simulink model "MdXX_RspOutComm"  (R2022b)
settings: Solver=FixedStepDiscrete  StartTime=0.0  StopTime=10.0  FixedStep=0.01  RelTol=1e-3
undefined symbols (not defined in the file or in its folder): KeSMSuRspStatHldTm_Val, MdRspLocal2, SrcReqTp1
libraries: simulink x64, RspLib x32
(part 4 of 5)

== system MdXX_RspOutComm/MdXX_RspOutCommCalc_Cal_sys/Subsystem/MdRspOutDataSelc13/BitSelector ==
  U : Inport
  Bit : Inport  Port=2
  Bitwise Operator : simulink/Logic and Bit Operations/Bitwise Operator  logicop=AND  UseBitMask=off  NumInputPorts=2  BitMask=bin2dec('11011001')  BitMaskRealWorld=Stored Integer
  Constant2 : Constant  OutDataTypeStr=uint32
  Constant4 : Constant  Value=0  OutDataTypeStr=uint32
  Relational Operator : RelationalOperator  Operator=>  OutDataTypeStr=boolean  RndMeth=Simplest  InputSameDT=off
  Shift Arithmetic : ArithShift  BitShiftNumberSource=Input port  BitShiftNumber=8  BitShiftDirection=Left
      settings: InputPortMap=u0,p1
  BitOut : Outport  VectorParamsAs1DForOutWhenUnconnected=off
  wires:
  Relational Operator/1 -> BitOut/1
  Constant4/1 -> Relational Operator/2
  Constant2/1 -> Shift Arithmetic/1
  Bitwise Operator/1 -> Relational Operator/1
  U/1 -> Bitwise Operator/1
  Shift Arithmetic/1 -> Bitwise Operator/2
  Bit/1 -> Shift Arithmetic/2

== system MdXX_RspOutComm/MdXX_RspOutCommCalc_Cal_sys/Subsystem/MdRspOutDataSelc13/BitSelector1 ==
  U : Inport
  Bit : Inport  Port=2
  Bitwise Operator : simulink/Logic and Bit Operations/Bitwise Operator  logicop=AND  UseBitMask=off  NumInputPorts=2  BitMask=bin2dec('11011001')  BitMaskRealWorld=Stored Integer
  Constant2 : Constant  OutDataTypeStr=uint32
  Constant4 : Constant  Value=0  OutDataTypeStr=uint32
  Relational Operator : RelationalOperator  Operator=>  OutDataTypeStr=boolean  RndMeth=Simplest  InputSameDT=off
  Shift Arithmetic : ArithShift  BitShiftNumberSource=Input port  BitShiftNumber=8  BitShiftDirection=Left
      settings: InputPortMap=u0,p1
  BitOut : Outport  VectorParamsAs1DForOutWhenUnconnected=off
  wires:
  Bit/1 -> Shift Arithmetic/2
  Shift Arithmetic/1 -> Bitwise Operator/2
  U/1 -> Bitwise Operator/1
  Bitwise Operator/1 -> Relational Operator/1
  Constant2/1 -> Shift Arithmetic/1
  Constant4/1 -> Relational Operator/2
  Relational Operator/1 -> BitOut/1

== system MdXX_RspOutComm/MdXX_RspOutCommCalc_Cal_sys/Subsystem/MdRspOutDataSelc14/BitSelector ==
  U : Inport
  Bit : Inport  Port=2
  Bitwise Operator : simulink/Logic and Bit Operations/Bitwise Operator  logicop=AND  UseBitMask=off  NumInputPorts=2  BitMask=bin2dec('11011001')  BitMaskRealWorld=Stored Integer
  Constant2 : Constant  OutDataTypeStr=uint32
  Constant4 : Constant  Value=0  OutDataTypeStr=uint32
  Relational Operator : RelationalOperator  Operator=>  OutDataTypeStr=boolean  RndMeth=Simplest  InputSameDT=off
  Shift Arithmetic : ArithShift  BitShiftNumberSource=Input port  BitShiftNumber=8  BitShiftDirection=Left
      settings: InputPortMap=u0,p1
  BitOut : Outport  VectorParamsAs1DForOutWhenUnconnected=off
  wires:
  Bit/1 -> Shift Arithmetic/2
  Shift Arithmetic/1 -> Bitwise Operator/2
  U/1 -> Bitwise Operator/1
  Bitwise Operator/1 -> Relational Operator/1
  Constant2/1 -> Shift Arithmetic/1
  Constant4/1 -> Relational Operator/2
  Relational Operator/1 -> BitOut/1

== system MdXX_RspOutComm/MdXX_RspOutCommCalc_Cal_sys/Subsystem/MdRspOutDataSelc14/BitSelector1 ==
  U : Inport
  Bit : Inport  Port=2
  Bitwise Operator : simulink/Logic and Bit Operations/Bitwise Operator  logicop=AND  UseBitMask=off  NumInputPorts=2  BitMask=bin2dec('11011001')  BitMaskRealWorld=Stored Integer
  Constant2 : Constant  OutDataTypeStr=uint32
  Constant4 : Constant  Value=0  OutDataTypeStr=uint32
  Relational Operator : RelationalOperator  Operator=>  OutDataTypeStr=boolean  RndMeth=Simplest  InputSameDT=off
  Shift Arithmetic : ArithShift  BitShiftNumberSource=Input port  BitShiftNumber=8  BitShiftDirection=Left
      settings: InputPortMap=u0,p1
  BitOut : Outport  VectorParamsAs1DForOutWhenUnconnected=off
  wires:
  Relational Operator/1 -> BitOut/1
  Constant4/1 -> Relational Operator/2
  Constant2/1 -> Shift Arithmetic/1
  Bitwise Operator/1 -> Relational Operator/1
  U/1 -> Bitwise Operator/1
  Shift Arithmetic/1 -> Bitwise Operator/2
  Bit/1 -> Shift Arithmetic/2

== system MdXX_RspOutComm/MdXX_RspOutCommCalc_Cal_sys/Subsystem/MdRspOutDataSelc15/BitSelector ==
  U : Inport
  Bit : Inport  Port=2
  Bitwise Operator : simulink/Logic and Bit Operations/Bitwise Operator  logicop=AND  UseBitMask=off  NumInputPorts=2  BitMask=bin2dec('11011001')  BitMaskRealWorld=Stored Integer
  Constant2 : Constant  OutDataTypeStr=uint32
  Constant4 : Constant  Value=0  OutDataTypeStr=uint32
  Relational Operator : RelationalOperator  Operator=>  OutDataTypeStr=boolean  RndMeth=Simplest  InputSameDT=off
  Shift Arithmetic : ArithShift  BitShiftNumberSource=Input port  BitShiftNumber=8  BitShiftDirection=Left
      settings: InputPortMap=u0,p1
  BitOut : Outport  VectorParamsAs1DForOutWhenUnconnected=off
  wires:
  Relational Operator/1 -> BitOut/1
  Constant4/1 -> Relational Operator/2
  Constant2/1 -> Shift Arithmetic/1
  Bitwise Operator/1 -> Relational Operator/1
  U/1 -> Bitwise Operator/1
  Shift Arithmetic/1 -> Bitwise Operator/2
  Bit/1 -> Shift Arithmetic/2

== system MdXX_RspOutComm/MdXX_RspOutCommCalc_Cal_sys/Subsystem/MdRspOutDataSelc15/BitSelector1 ==
  U : Inport
  Bit : Inport  Port=2
  Bitwise Operator : simulink/Logic and Bit Operations/Bitwise Operator  logicop=AND  UseBitMask=off  NumInputPorts=2  BitMask=bin2dec('11011001')  BitMaskRealWorld=Stored Integer
  Constant2 : Constant  OutDataTypeStr=uint32
  Constant4 : Constant  Value=0  OutDataTypeStr=uint32
  Relational Operator : RelationalOperator  Operator=>  OutDataTypeStr=boolean  RndMeth=Simplest  InputSameDT=off
  Shift Arithmetic : ArithShift  BitShiftNumberSource=Input port  BitShiftNumber=8  BitShiftDirection=Left
      settings: InputPortMap=u0,p1
  BitOut : Outport  VectorParamsAs1DForOutWhenUnconnected=off
  wires:
  Bit/1 -> Shift Arithmetic/2
  Shift Arithmetic/1 -> Bitwise Operator/2
  U/1 -> Bitwise Operator/1
  Bitwise Operator/1 -> Relational Operator/1
  Constant2/1 -> Shift Arithmetic/1
  Constant4/1 -> Relational Operator/2
  Relational Operator/1 -> BitOut/1

== system MdXX_RspOutComm/MdXX_RspOutCommCalc_Cal_sys/Subsystem/MdRspOutDataSelc16/BitSelector ==
  U : Inport
  Bit : Inport  Port=2
  Bitwise Operator : simulink/Logic and Bit Operations/Bitwise Operator  logicop=AND  UseBitMask=off  NumInputPorts=2  BitMask=bin2dec('11011001')  BitMaskRealWorld=Stored Integer
  Constant2 : Constant  OutDataTypeStr=uint32
  Constant4 : Constant  Value=0  OutDataTypeStr=uint32
  Relational Operator : RelationalOperator  Operator=>  OutDataTypeStr=boolean  RndMeth=Simplest  InputSameDT=off
  Shift Arithmetic : ArithShift  BitShiftNumberSource=Input port  BitShiftNumber=8  BitShiftDirection=Left
      settings: InputPortMap=u0,p1
  BitOut : Outport  VectorParamsAs1DForOutWhenUnconnected=off
  wires:
  Bit/1 -> Shift Arithmetic/2
  Shift Arithmetic/1 -> Bitwise Operator/2
  U/1 -> Bitwise Operator/1
  Bitwise Operator/1 -> Relational Operator/1
  Constant2/1 -> Shift Arithmetic/1
  Constant4/1 -> Relational Operator/2
  Relational Operator/1 -> BitOut/1

== system MdXX_RspOutComm/MdXX_RspOutCommCalc_Cal_sys/Subsystem/MdRspOutDataSelc16/BitSelector1 ==
  U : Inport
  Bit : Inport  Port=2
  Bitwise Operator : simulink/Logic and Bit Operations/Bitwise Operator  logicop=AND  UseBitMask=off  NumInputPorts=2  BitMask=bin2dec('11011001')  BitMaskRealWorld=Stored Integer
  Constant2 : Constant  OutDataTypeStr=uint32
  Constant4 : Constant  Value=0  OutDataTypeStr=uint32
  Relational Operator : RelationalOperator  Operator=>  OutDataTypeStr=boolean  RndMeth=Simplest  InputSameDT=off
  Shift Arithmetic : ArithShift  BitShiftNumberSource=Input port  BitShiftNumber=8  BitShiftDirection=Left
      settings: InputPortMap=u0,p1
  BitOut : Outport  VectorParamsAs1DForOutWhenUnconnected=off
  wires:
  Relational Operator/1 -> BitOut/1
  Constant4/1 -> Relational Operator/2
  Constant2/1 -> Shift Arithmetic/1
  Bitwise Operator/1 -> Relational Operator/1
  U/1 -> Bitwise Operator/1
  Shift Arithmetic/1 -> Bitwise Operator/2
  Bit/1 -> Shift Arithmetic/2

== system MdXX_RspOutComm/MdXX_RspOutCommCalc_Cal_sys/Subsystem/MdRspOutDataSelc17/BitSelector ==
  U : Inport
  Bit : Inport  Port=2
  Bitwise Operator : simulink/Logic and Bit Operations/Bitwise Operator  logicop=AND  UseBitMask=off  NumInputPorts=2  BitMask=bin2dec('11011001')  BitMaskRealWorld=Stored Integer
  Constant2 : Constant  OutDataTypeStr=uint32
  Constant4 : Constant  Value=0  OutDataTypeStr=uint32
  Relational Operator : RelationalOperator  Operator=>  OutDataTypeStr=boolean  RndMeth=Simplest  InputSameDT=off
  Shift Arithmetic : ArithShift  BitShiftNumberSource=Input port  BitShiftNumber=8  BitShiftDirection=Left
      settings: InputPortMap=u0,p1
  BitOut : Outport  VectorParamsAs1DForOutWhenUnconnected=off
  wires:
  Relational Operator/1 -> BitOut/1
  Constant4/1 -> Relational Operator/2
  Constant2/1 -> Shift Arithmetic/1
  Bitwise Operator/1 -> Relational Operator/1
  U/1 -> Bitwise Operator/1
  Shift Arithmetic/1 -> Bitwise Operator/2
  Bit/1 -> Shift Arithmetic/2

== system MdXX_RspOutComm/MdXX_RspOutCommCalc_Cal_sys/Subsystem/MdRspOutDataSelc17/BitSelector1 ==
  U : Inport
  Bit : Inport  Port=2
  Bitwise Operator : simulink/Logic and Bit Operations/Bitwise Operator  logicop=AND  UseBitMask=off  NumInputPorts=2  BitMask=bin2dec('11011001')  BitMaskRealWorld=Stored Integer
  Constant2 : Constant  OutDataTypeStr=uint32
  Constant4 : Constant  Value=0  OutDataTypeStr=uint32
  Relational Operator : RelationalOperator  Operator=>  OutDataTypeStr=boolean  RndMeth=Simplest  InputSameDT=off
  Shift Arithmetic : ArithShift  BitShiftNumberSource=Input port  BitShiftNumber=8  BitShiftDirection=Left
      settings: InputPortMap=u0,p1
  BitOut : Outport  VectorParamsAs1DForOutWhenUnconnected=off
  wires:
  Bit/1 -> Shift Arithmetic/2
  Shift Arithmetic/1 -> Bitwise Operator/2
  U/1 -> Bitwise Operator/1
  Bitwise Operator/1 -> Relational Operator/1
  Constant2/1 -> Shift Arithmetic/1
  Constant4/1 -> Relational Operator/2
  Relational Operator/1 -> BitOut/1

== system MdXX_RspOutComm/MdXX_RspOutCommCalc_Cal_sys/Subsystem/MdRspOutDataSelc18/BitSelector ==
  U : Inport
  Bit : Inport  Port=2
  Bitwise Operator : simulink/Logic and Bit Operations/Bitwise Operator  logicop=AND  UseBitMask=off  NumInputPorts=2  BitMask=bin2dec('11011001')  BitMaskRealWorld=Stored Integer
  Constant2 : Constant  OutDataTypeStr=uint32
  Constant4 : Constant  Value=0  OutDataTypeStr=uint32
  Relational Operator : RelationalOperator  Operator=>  OutDataTypeStr=boolean  RndMeth=Simplest  InputSameDT=off
  Shift Arithmetic : ArithShift  BitShiftNumberSource=Input port  BitShiftNumber=8  BitShiftDirection=Left
      settings: InputPortMap=u0,p1
  BitOut : Outport  VectorParamsAs1DForOutWhenUnconnected=off
  wires:
  Bit/1 -> Shift Arithmetic/2
  Shift Arithmetic/1 -> Bitwise Operator/2
  U/1 -> Bitwise Operator/1
  Bitwise Operator/1 -> Relational Operator/1
  Constant2/1 -> Shift Arithmetic/1
  Constant4/1 -> Relational Operator/2
  Relational Operator/1 -> BitOut/1

== system MdXX_RspOutComm/MdXX_RspOutCommCalc_Cal_sys/Subsystem/MdRspOutDataSelc18/BitSelector1 ==
  U : Inport
  Bit : Inport  Port=2
  Bitwise Operator : simulink/Logic and Bit Operations/Bitwise Operator  logicop=AND  UseBitMask=off  NumInputPorts=2  BitMask=bin2dec('11011001')  BitMaskRealWorld=Stored Integer
  Constant2 : Constant  OutDataTypeStr=uint32
  Constant4 : Constant  Value=0  OutDataTypeStr=uint32
  Relational Operator : RelationalOperator  Operator=>  OutDataTypeStr=boolean  RndMeth=Simplest  InputSameDT=off
  Shift Arithmetic : ArithShift  BitShiftNumberSource=Input port  BitShiftNumber=8  BitShiftDirection=Left
      settings: InputPortMap=u0,p1
  BitOut : Outport  VectorParamsAs1DForOutWhenUnconnected=off
  wires:
  Relational Operator/1 -> BitOut/1
  Constant4/1 -> Relational Operator/2
  Constant2/1 -> Shift Arithmetic/1
  Bitwise Operator/1 -> Relational Operator/1
  U/1 -> Bitwise Operator/1
  Shift Arithmetic/1 -> Bitwise Operator/2
  Bit/1 -> Shift Arithmetic/2

== system MdXX_RspOutComm/MdXX_RspOutCommCalc_Cal_sys/Subsystem/MdRspOutDataSelc19/BitSelector ==
  U : Inport
  Bit : Inport  Port=2
  Bitwise Operator : simulink/Logic and Bit Operations/Bitwise Operator  logicop=AND  UseBitMask=off  NumInputPorts=2  BitMask=bin2dec('11011001')  BitMaskRealWorld=Stored Integer
  Constant2 : Constant  OutDataTypeStr=uint32
  Constant4 : Constant  Value=0  OutDataTypeStr=uint32
  Relational Operator : RelationalOperator  Operator=>  OutDataTypeStr=boolean  RndMeth=Simplest  InputSameDT=off
  Shift Arithmetic : ArithShift  BitShiftNumberSource=Input port  BitShiftNumber=8  BitShiftDirection=Left
      settings: InputPortMap=u0,p1
  BitOut : Outport  VectorParamsAs1DForOutWhenUnconnected=off
  wires:
  Relational Operator/1 -> BitOut/1
  Constant4/1 -> Relational Operator/2
  Constant2/1 -> Shift Arithmetic/1
  Bitwise Operator/1 -> Relational Operator/1
  U/1 -> Bitwise Operator/1
  Shift Arithmetic/1 -> Bitwise Operator/2
  Bit/1 -> Shift Arithmetic/2

== system MdXX_RspOutComm/MdXX_RspOutCommCalc_Cal_sys/Subsystem/MdRspOutDataSelc19/BitSelector1 ==
  U : Inport
  Bit : Inport  Port=2
  Bitwise Operator : simulink/Logic and Bit Operations/Bitwise Operator  logicop=AND  UseBitMask=off  NumInputPorts=2  BitMask=bin2dec('11011001')  BitMaskRealWorld=Stored Integer
  Constant2 : Constant  OutDataTypeStr=uint32
  Constant4 : Constant  Value=0  OutDataTypeStr=uint32
  Relational Operator : RelationalOperator  Operator=>  OutDataTypeStr=boolean  RndMeth=Simplest  InputSameDT=off
  Shift Arithmetic : ArithShift  BitShiftNumberSource=Input port  BitShiftNumber=8  BitShiftDirection=Left
      settings: InputPortMap=u0,p1
  BitOut : Outport  VectorParamsAs1DForOutWhenUnconnected=off
  wires:
  Bit/1 -> Shift Arithmetic/2
  Shift Arithmetic/1 -> Bitwise Operator/2
  U/1 -> Bitwise Operator/1
  Bitwise Operator/1 -> Relational Operator/1
  Constant2/1 -> Shift Arithmetic/1
  Constant4/1 -> Relational Operator/2
  Relational Operator/1 -> BitOut/1

== system MdXX_RspOutComm/MdXX_RspOutCommCalc_Cal_sys/Subsystem/MdRspOutDataSelc2/BitSelector ==
  U : Inport
  Bit : Inport  Port=2
  Bitwise Operator : simulink/Logic and Bit Operations/Bitwise Operator  logicop=AND  UseBitMask=off  NumInputPorts=2  BitMask=bin2dec('11011001')  BitMaskRealWorld=Stored Integer
  Constant2 : Constant  OutDataTypeStr=uint32
  Constant4 : Constant  Value=0  OutDataTypeStr=uint32
  Relational Operator : RelationalOperator  Operator=>  OutDataTypeStr=boolean  RndMeth=Simplest  InputSameDT=off
  Shift Arithmetic : ArithShift  BitShiftNumberSource=Input port  BitShiftNumber=8  BitShiftDirection=Left
      settings: InputPortMap=u0,p1
  BitOut : Outport  VectorParamsAs1DForOutWhenUnconnected=off
  wires:
  Bit/1 -> Shift Arithmetic/2
  Shift Arithmetic/1 -> Bitwise Operator/2
  U/1 -> Bitwise Operator/1
  Bitwise Operator/1 -> Relational Operator/1
  Constant2/1 -> Shift Arithmetic/1
  Constant4/1 -> Relational Operator/2
  Relational Operator/1 -> BitOut/1

== system MdXX_RspOutComm/MdXX_RspOutCommCalc_Cal_sys/Subsystem/MdRspOutDataSelc2/BitSelector1 ==
  U : Inport
  Bit : Inport  Port=2
  Bitwise Operator : simulink/Logic and Bit Operations/Bitwise Operator  logicop=AND  UseBitMask=off  NumInputPorts=2  BitMask=bin2dec('11011001')  BitMaskRealWorld=Stored Integer
  Constant2 : Constant  OutDataTypeStr=uint32
  Constant4 : Constant  Value=0  OutDataTypeStr=uint32
  Relational Operator : RelationalOperator  Operator=>  OutDataTypeStr=boolean  RndMeth=Simplest  InputSameDT=off
  Shift Arithmetic : ArithShift  BitShiftNumberSource=Input port  BitShiftNumber=8  BitShiftDirection=Left
      settings: InputPortMap=u0,p1
  BitOut : Outport  VectorParamsAs1DForOutWhenUnconnected=off
  wires:
  Relational Operator/1 -> BitOut/1
  Constant4/1 -> Relational Operator/2
  Constant2/1 -> Shift Arithmetic/1
  Bitwise Operator/1 -> Relational Operator/1
  U/1 -> Bitwise Operator/1
  Shift Arithmetic/1 -> Bitwise Operator/2
  Bit/1 -> Shift Arithmetic/2

== system MdXX_RspOutComm/MdXX_RspOutCommCalc_Cal_sys/Subsystem/MdRspOutDataSelc20/BitSelector ==
  U : Inport
  Bit : Inport  Port=2
  Bitwise Operator : simulink/Logic and Bit Operations/Bitwise Operator  logicop=AND  UseBitMask=off  NumInputPorts=2  BitMask=bin2dec('11011001')  BitMaskRealWorld=Stored Integer
  Constant2 : Constant  OutDataTypeStr=uint32
  Constant4 : Constant  Value=0  OutDataTypeStr=uint32
  Relational Operator : RelationalOperator  Operator=>  OutDataTypeStr=boolean  RndMeth=Simplest  InputSameDT=off
  Shift Arithmetic : ArithShift  BitShiftNumberSource=Input port  BitShiftNumber=8  BitShiftDirection=Left
      settings: InputPortMap=u0,p1
  BitOut : Outport  VectorParamsAs1DForOutWhenUnconnected=off
  wires:
  Bit/1 -> Shift Arithmetic/2
  Shift Arithmetic/1 -> Bitwise Operator/2
  U/1 -> Bitwise Operator/1
  Bitwise Operator/1 -> Relational Operator/1
  Constant2/1 -> Shift Arithmetic/1
  Constant4/1 -> Relational Operator/2
  Relational Operator/1 -> BitOut/1

== system MdXX_RspOutComm/MdXX_RspOutCommCalc_Cal_sys/Subsystem/MdRspOutDataSelc20/BitSelector1 ==
  U : Inport
  Bit : Inport  Port=2
  Bitwise Operator : simulink/Logic and Bit Operations/Bitwise Operator  logicop=AND  UseBitMask=off  NumInputPorts=2  BitMask=bin2dec('11011001')  BitMaskRealWorld=Stored Integer
  Constant2 : Constant  OutDataTypeStr=uint32
  Constant4 : Constant  Value=0  OutDataTypeStr=uint32
  Relational Operator : RelationalOperator  Operator=>  OutDataTypeStr=boolean  RndMeth=Simplest  InputSameDT=off
  Shift Arithmetic : ArithShift  BitShiftNumberSource=Input port  BitShiftNumber=8  BitShiftDirection=Left
      settings: InputPortMap=u0,p1
  BitOut : Outport  VectorParamsAs1DForOutWhenUnconnected=off
  wires:
  Relational Operator/1 -> BitOut/1
  Constant4/1 -> Relational Operator/2
  Constant2/1 -> Shift Arithmetic/1
  Bitwise Operator/1 -> Relational Operator/1
  U/1 -> Bitwise Operator/1
  Shift Arithmetic/1 -> Bitwise Operator/2
  Bit/1 -> Shift Arithmetic/2

== system MdXX_RspOutComm/MdXX_RspOutCommCalc_Cal_sys/Subsystem/MdRspOutDataSelc21/BitSelector ==
  U : Inport
  Bit : Inport  Port=2
  Bitwise Operator : simulink/Logic and Bit Operations/Bitwise Operator  logicop=AND  UseBitMask=off  NumInputPorts=2  BitMask=bin2dec('11011001')  BitMaskRealWorld=Stored Integer
  Constant2 : Constant  OutDataTypeStr=uint32
  Constant4 : Constant  Value=0  OutDataTypeStr=uint32
  Relational Operator : RelationalOperator  Operator=>  OutDataTypeStr=boolean  RndMeth=Simplest  InputSameDT=off
  Shift Arithmetic : ArithShift  BitShiftNumberSource=Input port  BitShiftNumber=8  BitShiftDirection=Left
      settings: InputPortMap=u0,p1
  BitOut : Outport  VectorParamsAs1DForOutWhenUnconnected=off
  wires:
  Relational Operator/1 -> BitOut/1
  Constant4/1 -> Relational Operator/2
  Constant2/1 -> Shift Arithmetic/1
  Bitwise Operator/1 -> Relational Operator/1
  U/1 -> Bitwise Operator/1
  Shift Arithmetic/1 -> Bitwise Operator/2
  Bit/1 -> Shift Arithmetic/2

== system MdXX_RspOutComm/MdXX_RspOutCommCalc_Cal_sys/Subsystem/MdRspOutDataSelc21/BitSelector1 ==
  U : Inport
  Bit : Inport  Port=2
  Bitwise Operator : simulink/Logic and Bit Operations/Bitwise Operator  logicop=AND  UseBitMask=off  NumInputPorts=2  BitMask=bin2dec('11011001')  BitMaskRealWorld=Stored Integer
  Constant2 : Constant  OutDataTypeStr=uint32
  Constant4 : Constant  Value=0  OutDataTypeStr=uint32
  Relational Operator : RelationalOperator  Operator=>  OutDataTypeStr=boolean  RndMeth=Simplest  InputSameDT=off
  Shift Arithmetic : ArithShift  BitShiftNumberSource=Input port  BitShiftNumber=8  BitShiftDirection=Left
      settings: InputPortMap=u0,p1
  BitOut : Outport  VectorParamsAs1DForOutWhenUnconnected=off
  wires:
  Bit/1 -> Shift Arithmetic/2
  Shift Arithmetic/1 -> Bitwise Operator/2
  U/1 -> Bitwise Operator/1
  Bitwise Operator/1 -> Relational Operator/1
  Constant2/1 -> Shift Arithmetic/1
  Constant4/1 -> Relational Operator/2
  Relational Operator/1 -> BitOut/1

== system MdXX_RspOutComm/MdXX_RspOutCommCalc_Cal_sys/Subsystem/MdRspOutDataSelc22/BitSelector ==
  U : Inport
  Bit : Inport  Port=2
  Bitwise Operator : simulink/Logic and Bit Operations/Bitwise Operator  logicop=AND  UseBitMask=off  NumInputPorts=2  BitMask=bin2dec('11011001')  BitMaskRealWorld=Stored Integer
  Constant2 : Constant  OutDataTypeStr=uint32
  Constant4 : Constant  Value=0  OutDataTypeStr=uint32
  Relational Operator : RelationalOperator  Operator=>  OutDataTypeStr=boolean  RndMeth=Simplest  InputSameDT=off
  Shift Arithmetic : ArithShift  BitShiftNumberSource=Input port  BitShiftNumber=8  BitShiftDirection=Left
      settings: InputPortMap=u0,p1
  BitOut : Outport  VectorParamsAs1DForOutWhenUnconnected=off
  wires:
  Bit/1 -> Shift Arithmetic/2
  Shift Arithmetic/1 -> Bitwise Operator/2
  U/1 -> Bitwise Operator/1
  Bitwise Operator/1 -> Relational Operator/1
  Constant2/1 -> Shift Arithmetic/1
  Constant4/1 -> Relational Operator/2
  Relational Operator/1 -> BitOut/1

== system MdXX_RspOutComm/MdXX_RspOutCommCalc_Cal_sys/Subsystem/MdRspOutDataSelc22/BitSelector1 ==
  U : Inport
  Bit : Inport  Port=2
  Bitwise Operator : simulink/Logic and Bit Operations/Bitwise Operator  logicop=AND  UseBitMask=off  NumInputPorts=2  BitMask=bin2dec('11011001')  BitMaskRealWorld=Stored Integer
  Constant2 : Constant  OutDataTypeStr=uint32
  Constant4 : Constant  Value=0  OutDataTypeStr=uint32
  Relational Operator : RelationalOperator  Operator=>  OutDataTypeStr=boolean  RndMeth=Simplest  InputSameDT=off
  Shift Arithmetic : ArithShift  BitShiftNumberSource=Input port  BitShiftNumber=8  BitShiftDirection=Left
      settings: InputPortMap=u0,p1
  BitOut : Outport  VectorParamsAs1DForOutWhenUnconnected=off
  wires:
  Relational Operator/1 -> BitOut/1
  Constant4/1 -> Relational Operator/2
  Constant2/1 -> Shift Arithmetic/1
  Bitwise Operator/1 -> Relational Operator/1
  U/1 -> Bitwise Operator/1
  Shift Arithmetic/1 -> Bitwise Operator/2
  Bit/1 -> Shift Arithmetic/2

== system MdXX_RspOutComm/MdXX_RspOutCommCalc_Cal_sys/Subsystem/MdRspOutDataSelc23/BitSelector ==
  U : Inport
  Bit : Inport  Port=2
  Bitwise Operator : simulink/Logic and Bit Operations/Bitwise Operator  logicop=AND  UseBitMask=off  NumInputPorts=2  BitMask=bin2dec('11011001')  BitMaskRealWorld=Stored Integer
  Constant2 : Constant  OutDataTypeStr=uint32
  Constant4 : Constant  Value=0  OutDataTypeStr=uint32
  Relational Operator : RelationalOperator  Operator=>  OutDataTypeStr=boolean  RndMeth=Simplest  InputSameDT=off
  Shift Arithmetic : ArithShift  BitShiftNumberSource=Input port  BitShiftNumber=8  BitShiftDirection=Left
      settings: InputPortMap=u0,p1
  BitOut : Outport  VectorParamsAs1DForOutWhenUnconnected=off
  wires:
  Relational Operator/1 -> BitOut/1
  Constant4/1 -> Relational Operator/2
  Constant2/1 -> Shift Arithmetic/1
  Bitwise Operator/1 -> Relational Operator/1
  U/1 -> Bitwise Operator/1
  Shift Arithmetic/1 -> Bitwise Operator/2
  Bit/1 -> Shift Arithmetic/2

== system MdXX_RspOutComm/MdXX_RspOutCommCalc_Cal_sys/Subsystem/MdRspOutDataSelc23/BitSelector1 ==
  U : Inport
  Bit : Inport  Port=2
  Bitwise Operator : simulink/Logic and Bit Operations/Bitwise Operator  logicop=AND  UseBitMask=off  NumInputPorts=2  BitMask=bin2dec('11011001')  BitMaskRealWorld=Stored Integer
  Constant2 : Constant  OutDataTypeStr=uint32
  Constant4 : Constant  Value=0  OutDataTypeStr=uint32
  Relational Operator : RelationalOperator  Operator=>  OutDataTypeStr=boolean  RndMeth=Simplest  InputSameDT=off
  Shift Arithmetic : ArithShift  BitShiftNumberSource=Input port  BitShiftNumber=8  BitShiftDirection=Left
      settings: InputPortMap=u0,p1
  BitOut : Outport  VectorParamsAs1DForOutWhenUnconnected=off
  wires:
  Bit/1 -> Shift Arithmetic/2
  Shift Arithmetic/1 -> Bitwise Operator/2
  U/1 -> Bitwise Operator/1
  Bitwise Operator/1 -> Relational Operator/1
  Constant2/1 -> Shift Arithmetic/1
  Constant4/1 -> Relational Operator/2
  Relational Operator/1 -> BitOut/1

== system MdXX_RspOutComm/MdXX_RspOutCommCalc_Cal_sys/Subsystem/MdRspOutDataSelc24/BitSelector ==
  U : Inport
  Bit : Inport  Port=2
  Bitwise Operator : simulink/Logic and Bit Operations/Bitwise Operator  logicop=AND  UseBitMask=off  NumInputPorts=2  BitMask=bin2dec('11011001')  BitMaskRealWorld=Stored Integer
  Constant2 : Constant  OutDataTypeStr=uint32
  Constant4 : Constant  Value=0  OutDataTypeStr=uint32
  Relational Operator : RelationalOperator  Operator=>  OutDataTypeStr=boolean  RndMeth=Simplest  InputSameDT=off
  Shift Arithmetic : ArithShift  BitShiftNumberSource=Input port  BitShiftNumber=8  BitShiftDirection=Left
      settings: InputPortMap=u0,p1
  BitOut : Outport  VectorParamsAs1DForOutWhenUnconnected=off
  wires:
  Bit/1 -> Shift Arithmetic/2
  Shift Arithmetic/1 -> Bitwise Operator/2
  U/1 -> Bitwise Operator/1
  Bitwise Operator/1 -> Relational Operator/1
  Constant2/1 -> Shift Arithmetic/1
  Constant4/1 -> Relational Operator/2
  Relational Operator/1 -> BitOut/1

== system MdXX_RspOutComm/MdXX_RspOutCommCalc_Cal_sys/Subsystem/MdRspOutDataSelc24/BitSelector1 ==
  U : Inport
  Bit : Inport  Port=2
  Bitwise Operator : simulink/Logic and Bit Operations/Bitwise Operator  logicop=AND  UseBitMask=off  NumInputPorts=2  BitMask=bin2dec('11011001')  BitMaskRealWorld=Stored Integer
  Constant2 : Constant  OutDataTypeStr=uint32
  Constant4 : Constant  Value=0  OutDataTypeStr=uint32
  Relational Operator : RelationalOperator  Operator=>  OutDataTypeStr=boolean  RndMeth=Simplest  InputSameDT=off
  Shift Arithmetic : ArithShift  BitShiftNumberSource=Input port  BitShiftNumber=8  BitShiftDirection=Left
      settings: InputPortMap=u0,p1
  BitOut : Outport  VectorParamsAs1DForOutWhenUnconnected=off
  wires:
  Relational Operator/1 -> BitOut/1
  Constant4/1 -> Relational Operator/2
  Constant2/1 -> Shift Arithmetic/1
  Bitwise Operator/1 -> Relational Operator/1
  U/1 -> Bitwise Operator/1
  Shift Arithmetic/1 -> Bitwise Operator/2
  Bit/1 -> Shift Arithmetic/2

== system MdXX_RspOutComm/MdXX_RspOutCommCalc_Cal_sys/Subsystem/MdRspOutDataSelc25/BitSelector ==
  U : Inport
  Bit : Inport  Port=2
  Bitwise Operator : simulink/Logic and Bit Operations/Bitwise Operator  logicop=AND  UseBitMask=off  NumInputPorts=2  BitMask=bin2dec('11011001')  BitMaskRealWorld=Stored Integer
  Constant2 : Constant  OutDataTypeStr=uint32
  Constant4 : Constant  Value=0  OutDataTypeStr=uint32
  Relational Operator : RelationalOperator  Operator=>  OutDataTypeStr=boolean  RndMeth=Simplest  InputSameDT=off
  Shift Arithmetic : ArithShift  BitShiftNumberSource=Input port  BitShiftNumber=8  BitShiftDirection=Left
      settings: InputPortMap=u0,p1
  BitOut : Outport  VectorParamsAs1DForOutWhenUnconnected=off
  wires:
  Relational Operator/1 -> BitOut/1
  Constant4/1 -> Relational Operator/2
  Constant2/1 -> Shift Arithmetic/1
  Bitwise Operator/1 -> Relational Operator/1
  U/1 -> Bitwise Operator/1
  Shift Arithmetic/1 -> Bitwise Operator/2
  Bit/1 -> Shift Arithmetic/2

== system MdXX_RspOutComm/MdXX_RspOutCommCalc_Cal_sys/Subsystem/MdRspOutDataSelc25/BitSelector1 ==
  U : Inport
  Bit : Inport  Port=2
  Bitwise Operator : simulink/Logic and Bit Operations/Bitwise Operator  logicop=AND  UseBitMask=off  NumInputPorts=2  BitMask=bin2dec('11011001')  BitMaskRealWorld=Stored Integer
  Constant2 : Constant  OutDataTypeStr=uint32
  Constant4 : Constant  Value=0  OutDataTypeStr=uint32
  Relational Operator : RelationalOperator  Operator=>  OutDataTypeStr=boolean  RndMeth=Simplest  InputSameDT=off
  Shift Arithmetic : ArithShift  BitShiftNumberSource=Input port  BitShiftNumber=8  BitShiftDirection=Left
      settings: InputPortMap=u0,p1
  BitOut : Outport  VectorParamsAs1DForOutWhenUnconnected=off
  wires:
  Bit/1 -> Shift Arithmetic/2
  Shift Arithmetic/1 -> Bitwise Operator/2
  U/1 -> Bitwise Operator/1
  Bitwise Operator/1 -> Relational Operator/1
  Constant2/1 -> Shift Arithmetic/1
  Constant4/1 -> Relational Operator/2
  Relational Operator/1 -> BitOut/1

== system MdXX_RspOutComm/MdXX_RspOutCommCalc_Cal_sys/Subsystem/MdRspOutDataSelc26/BitSelector ==
  U : Inport
  Bit : Inport  Port=2
  Bitwise Operator : simulink/Logic and Bit Operations/Bitwise Operator  logicop=AND  UseBitMask=off  NumInputPorts=2  BitMask=bin2dec('11011001')  BitMaskRealWorld=Stored Integer
  Constant2 : Constant  OutDataTypeStr=uint32
  Constant4 : Constant  Value=0  OutDataTypeStr=uint32
  Relational Operator : RelationalOperator  Operator=>  OutDataTypeStr=boolean  RndMeth=Simplest  InputSameDT=off
  Shift Arithmetic : ArithShift  BitShiftNumberSource=Input port  BitShiftNumber=8  BitShiftDirection=Left
      settings: InputPortMap=u0,p1
  BitOut : Outport  VectorParamsAs1DForOutWhenUnconnected=off
  wires:
  Bit/1 -> Shift Arithmetic/2
  Shift Arithmetic/1 -> Bitwise Operator/2
  U/1 -> Bitwise Operator/1
  Bitwise Operator/1 -> Relational Operator/1
  Constant2/1 -> Shift Arithmetic/1
  Constant4/1 -> Relational Operator/2
  Relational Operator/1 -> BitOut/1

== system MdXX_RspOutComm/MdXX_RspOutCommCalc_Cal_sys/Subsystem/MdRspOutDataSelc26/BitSelector1 ==
  U : Inport
  Bit : Inport  Port=2
  Bitwise Operator : simulink/Logic and Bit Operations/Bitwise Operator  logicop=AND  UseBitMask=off  NumInputPorts=2  BitMask=bin2dec('11011001')  BitMaskRealWorld=Stored Integer
  Constant2 : Constant  OutDataTypeStr=uint32
  Constant4 : Constant  Value=0  OutDataTypeStr=uint32
  Relational Operator : RelationalOperator  Operator=>  OutDataTypeStr=boolean  RndMeth=Simplest  InputSameDT=off
  Shift Arithmetic : ArithShift  BitShiftNumberSource=Input port  BitShiftNumber=8  BitShiftDirection=Left
      settings: InputPortMap=u0,p1
  BitOut : Outport  VectorParamsAs1DForOutWhenUnconnected=off
  wires:
  Relational Operator/1 -> BitOut/1
  Constant4/1 -> Relational Operator/2
  Constant2/1 -> Shift Arithmetic/1
  Bitwise Operator/1 -> Relational Operator/1
  U/1 -> Bitwise Operator/1
  Shift Arithmetic/1 -> Bitwise Operator/2
  Bit/1 -> Shift Arithmetic/2

== system MdXX_RspOutComm/MdXX_RspOutCommCalc_Cal_sys/Subsystem/MdRspOutDataSelc27/BitSelector ==
  U : Inport
  Bit : Inport  Port=2
  Bitwise Operator : simulink/Logic and Bit Operations/Bitwise Operator  logicop=AND  UseBitMask=off  NumInputPorts=2  BitMask=bin2dec('11011001')  BitMaskRealWorld=Stored Integer
  Constant2 : Constant  OutDataTypeStr=uint32
  Constant4 : Constant  Value=0  OutDataTypeStr=uint32
  Relational Operator : RelationalOperator  Operator=>  OutDataTypeStr=boolean  RndMeth=Simplest  InputSameDT=off
  Shift Arithmetic : ArithShift  BitShiftNumberSource=Input port  BitShiftNumber=8  BitShiftDirection=Left
      settings: InputPortMap=u0,p1
  BitOut : Outport  VectorParamsAs1DForOutWhenUnconnected=off
  wires:
  Relational Operator/1 -> BitOut/1
  Constant4/1 -> Relational Operator/2
  Constant2/1 -> Shift Arithmetic/1
  Bitwise Operator/1 -> Relational Operator/1
  U/1 -> Bitwise Operator/1
  Shift Arithmetic/1 -> Bitwise Operator/2
  Bit/1 -> Shift Arithmetic/2

== system MdXX_RspOutComm/MdXX_RspOutCommCalc_Cal_sys/Subsystem/MdRspOutDataSelc27/BitSelector1 ==
  U : Inport
  Bit : Inport  Port=2
  Bitwise Operator : simulink/Logic and Bit Operations/Bitwise Operator  logicop=AND  UseBitMask=off  NumInputPorts=2  BitMask=bin2dec('11011001')  BitMaskRealWorld=Stored Integer
  Constant2 : Constant  OutDataTypeStr=uint32
  Constant4 : Constant  Value=0  OutDataTypeStr=uint32
  Relational Operator : RelationalOperator  Operator=>  OutDataTypeStr=boolean  RndMeth=Simplest  InputSameDT=off
  Shift Arithmetic : ArithShift  BitShiftNumberSource=Input port  BitShiftNumber=8  BitShiftDirection=Left
      settings: InputPortMap=u0,p1
  BitOut : Outport  VectorParamsAs1DForOutWhenUnconnected=off
  wires:
  Bit/1 -> Shift Arithmetic/2
  Shift Arithmetic/1 -> Bitwise Operator/2
  U/1 -> Bitwise Operator/1
  Bitwise Operator/1 -> Relational Operator/1
  Constant2/1 -> Shift Arithmetic/1
  Constant4/1 -> Relational Operator/2
  Relational Operator/1 -> BitOut/1

== system MdXX_RspOutComm/MdXX_RspOutCommCalc_Cal_sys/Subsystem/MdRspOutDataSelc28/BitSelector ==
  U : Inport
  Bit : Inport  Port=2
  Bitwise Operator : simulink/Logic and Bit Operations/Bitwise Operator  logicop=AND  UseBitMask=off  NumInputPorts=2  BitMask=bin2dec('11011001')  BitMaskRealWorld=Stored Integer
  Constant2 : Constant  OutDataTypeStr=uint32
  Constant4 : Constant  Value=0  OutDataTypeStr=uint32
  Relational Operator : RelationalOperator  Operator=>  OutDataTypeStr=boolean  RndMeth=Simplest  InputSameDT=off
  Shift Arithmetic : ArithShift  BitShiftNumberSource=Input port  BitShiftNumber=8  BitShiftDirection=Left
      settings: InputPortMap=u0,p1
  BitOut : Outport  VectorParamsAs1DForOutWhenUnconnected=off
  wires:
  Bit/1 -> Shift Arithmetic/2
  Shift Arithmetic/1 -> Bitwise Operator/2
  U/1 -> Bitwise Operator/1
  Bitwise Operator/1 -> Relational Operator/1
  Constant2/1 -> Shift Arithmetic/1
  Constant4/1 -> Relational Operator/2
  Relational Operator/1 -> BitOut/1

== system MdXX_RspOutComm/MdXX_RspOutCommCalc_Cal_sys/Subsystem/MdRspOutDataSelc28/BitSelector1 ==
  U : Inport
  Bit : Inport  Port=2
  Bitwise Operator : simulink/Logic and Bit Operations/Bitwise Operator  logicop=AND  UseBitMask=off  NumInputPorts=2  BitMask=bin2dec('11011001')  BitMaskRealWorld=Stored Integer
  Constant2 : Constant  OutDataTypeStr=uint32
  Constant4 : Constant  Value=0  OutDataTypeStr=uint32
  Relational Operator : RelationalOperator  Operator=>  OutDataTypeStr=boolean  RndMeth=Simplest  InputSameDT=off
  Shift Arithmetic : ArithShift  BitShiftNumberSource=Input port  BitShiftNumber=8  BitShiftDirection=Left
      settings: InputPortMap=u0,p1
  BitOut : Outport  VectorParamsAs1DForOutWhenUnconnected=off
  wires:
  Relational Operator/1 -> BitOut/1
  Constant4/1 -> Relational Operator/2
  Constant2/1 -> Shift Arithmetic/1
  Bitwise Operator/1 -> Relational Operator/1
  U/1 -> Bitwise Operator/1
  Shift Arithmetic/1 -> Bitwise Operator/2
  Bit/1 -> Shift Arithmetic/2

== system MdXX_RspOutComm/MdXX_RspOutCommCalc_Cal_sys/Subsystem/MdRspOutDataSelc29/BitSelector ==
  U : Inport
  Bit : Inport  Port=2
  Bitwise Operator : simulink/Logic and Bit Operations/Bitwise Operator  logicop=AND  UseBitMask=off  NumInputPorts=2  BitMask=bin2dec('11011001')  BitMaskRealWorld=Stored Integer
  Constant2 : Constant  OutDataTypeStr=uint32
  Constant4 : Constant  Value=0  OutDataTypeStr=uint32
  Relational Operator : RelationalOperator  Operator=>  OutDataTypeStr=boolean  RndMeth=Simplest  InputSameDT=off
  Shift Arithmetic : ArithShift  BitShiftNumberSource=Input port  BitShiftNumber=8  BitShiftDirection=Left
      settings: InputPortMap=u0,p1
  BitOut : Outport  VectorParamsAs1DForOutWhenUnconnected=off
  wires:
  Relational Operator/1 -> BitOut/1
  Constant4/1 -> Relational Operator/2
  Constant2/1 -> Shift Arithmetic/1
  Bitwise Operator/1 -> Relational Operator/1
  U/1 -> Bitwise Operator/1
  Shift Arithmetic/1 -> Bitwise Operator/2
  Bit/1 -> Shift Arithmetic/2

== system MdXX_RspOutComm/MdXX_RspOutCommCalc_Cal_sys/Subsystem/MdRspOutDataSelc29/BitSelector1 ==
  U : Inport
  Bit : Inport  Port=2
  Bitwise Operator : simulink/Logic and Bit Operations/Bitwise Operator  logicop=AND  UseBitMask=off  NumInputPorts=2  BitMask=bin2dec('11011001')  BitMaskRealWorld=Stored Integer
  Constant2 : Constant  OutDataTypeStr=uint32
  Constant4 : Constant  Value=0  OutDataTypeStr=uint32
  Relational Operator : RelationalOperator  Operator=>  OutDataTypeStr=boolean  RndMeth=Simplest  InputSameDT=off
  Shift Arithmetic : ArithShift  BitShiftNumberSource=Input port  BitShiftNumber=8  BitShiftDirection=Left
      settings: InputPortMap=u0,p1
  BitOut : Outport  VectorParamsAs1DForOutWhenUnconnected=off
  wires:
  Bit/1 -> Shift Arithmetic/2
  Shift Arithmetic/1 -> Bitwise Operator/2
  U/1 -> Bitwise Operator/1
  Bitwise Operator/1 -> Relational Operator/1
  Constant2/1 -> Shift Arithmetic/1
  Constant4/1 -> Relational Operator/2
  Relational Operator/1 -> BitOut/1

== system MdXX_RspOutComm/MdXX_RspOutCommCalc_Cal_sys/Subsystem/MdRspOutDataSelc3/BitSelector ==
  U : Inport
  Bit : Inport  Port=2
  Bitwise Operator : simulink/Logic and Bit Operations/Bitwise Operator  logicop=AND  UseBitMask=off  NumInputPorts=2  BitMask=bin2dec('11011001')  BitMaskRealWorld=Stored Integer
  Constant2 : Constant  OutDataTypeStr=uint32
  Constant4 : Constant  Value=0  OutDataTypeStr=uint32
  Relational Operator : RelationalOperator  Operator=>  OutDataTypeStr=boolean  RndMeth=Simplest  InputSameDT=off
  Shift Arithmetic : ArithShift  BitShiftNumberSource=Input port  BitShiftNumber=8  BitShiftDirection=Left
      settings: InputPortMap=u0,p1
  BitOut : Outport  VectorParamsAs1DForOutWhenUnconnected=off
  wires:
  Relational Operator/1 -> BitOut/1
  Constant4/1 -> Relational Operator/2
  Constant2/1 -> Shift Arithmetic/1
  Bitwise Operator/1 -> Relational Operator/1
  U/1 -> Bitwise Operator/1
  Shift Arithmetic/1 -> Bitwise Operator/2
  Bit/1 -> Shift Arithmetic/2

== system MdXX_RspOutComm/MdXX_RspOutCommCalc_Cal_sys/Subsystem/MdRspOutDataSelc3/BitSelector1 ==
  U : Inport
  Bit : Inport  Port=2
  Bitwise Operator : simulink/Logic and Bit Operations/Bitwise Operator  logicop=AND  UseBitMask=off  NumInputPorts=2  BitMask=bin2dec('11011001')  BitMaskRealWorld=Stored Integer
  Constant2 : Constant  OutDataTypeStr=uint32
  Constant4 : Constant  Value=0  OutDataTypeStr=uint32
  Relational Operator : RelationalOperator  Operator=>  OutDataTypeStr=boolean  RndMeth=Simplest  InputSameDT=off
  Shift Arithmetic : ArithShift  BitShiftNumberSource=Input port  BitShiftNumber=8  BitShiftDirection=Left
      settings: InputPortMap=u0,p1
  BitOut : Outport  VectorParamsAs1DForOutWhenUnconnected=off
  wires:
  Bit/1 -> Shift Arithmetic/2
  Shift Arithmetic/1 -> Bitwise Operator/2
  U/1 -> Bitwise Operator/1
  Bitwise Operator/1 -> Relational Operator/1
  Constant2/1 -> Shift Arithmetic/1
  Constant4/1 -> Relational Operator/2
  Relational Operator/1 -> BitOut/1

== system MdXX_RspOutComm/MdXX_RspOutCommCalc_Cal_sys/Subsystem/MdRspOutDataSelc30/BitSelector ==
  U : Inport
  Bit : Inport  Port=2
  Bitwise Operator : simulink/Logic and Bit Operations/Bitwise Operator  logicop=AND  UseBitMask=off  NumInputPorts=2  BitMask=bin2dec('11011001')  BitMaskRealWorld=Stored Integer
  Constant2 : Constant  OutDataTypeStr=uint32
  Constant4 : Constant  Value=0  OutDataTypeStr=uint32
  Relational Operator : RelationalOperator  Operator=>  OutDataTypeStr=boolean  RndMeth=Simplest  InputSameDT=off
  Shift Arithmetic : ArithShift  BitShiftNumberSource=Input port  BitShiftNumber=8  BitShiftDirection=Left
      settings: InputPortMap=u0,p1
  BitOut : Outport  VectorParamsAs1DForOutWhenUnconnected=off
  wires:
  Bit/1 -> Shift Arithmetic/2
  Shift Arithmetic/1 -> Bitwise Operator/2
  U/1 -> Bitwise Operator/1
  Bitwise Operator/1 -> Relational Operator/1
  Constant2/1 -> Shift Arithmetic/1
  Constant4/1 -> Relational Operator/2
  Relational Operator/1 -> BitOut/1

== system MdXX_RspOutComm/MdXX_RspOutCommCalc_Cal_sys/Subsystem/MdRspOutDataSelc30/BitSelector1 ==
  U : Inport
  Bit : Inport  Port=2
  Bitwise Operator : simulink/Logic and Bit Operations/Bitwise Operator  logicop=AND  UseBitMask=off  NumInputPorts=2  BitMask=bin2dec('11011001')  BitMaskRealWorld=Stored Integer
  Constant2 : Constant  OutDataTypeStr=uint32
  Constant4 : Constant  Value=0  OutDataTypeStr=uint32
  Relational Operator : RelationalOperator  Operator=>  OutDataTypeStr=boolean  RndMeth=Simplest  InputSameDT=off
  Shift Arithmetic : ArithShift  BitShiftNumberSource=Input port  BitShiftNumber=8  BitShiftDirection=Left
      settings: InputPortMap=u0,p1
  BitOut : Outport  VectorParamsAs1DForOutWhenUnconnected=off
  wires:
  Relational Operator/1 -> BitOut/1
  Constant4/1 -> Relational Operator/2
  Constant2/1 -> Shift Arithmetic/1
  Bitwise Operator/1 -> Relational Operator/1
  U/1 -> Bitwise Operator/1
  Shift Arithmetic/1 -> Bitwise Operator/2
  Bit/1 -> Shift Arithmetic/2

== system MdXX_RspOutComm/MdXX_RspOutCommCalc_Cal_sys/Subsystem/MdRspOutDataSelc31/BitSelector ==
  U : Inport
  Bit : Inport  Port=2
  Bitwise Operator : simulink/Logic and Bit Operations/Bitwise Operator  logicop=AND  UseBitMask=off  NumInputPorts=2  BitMask=bin2dec('11011001')  BitMaskRealWorld=Stored Integer
  Constant2 : Constant  OutDataTypeStr=uint32
  Constant4 : Constant  Value=0  OutDataTypeStr=uint32
  Relational Operator : RelationalOperator  Operator=>  OutDataTypeStr=boolean  RndMeth=Simplest  InputSameDT=off
  Shift Arithmetic : ArithShift  BitShiftNumberSource=Input port  BitShiftNumber=8  BitShiftDirection=Left
      settings: InputPortMap=u0,p1
  BitOut : Outport  VectorParamsAs1DForOutWhenUnconnected=off
  wires:
  Relational Operator/1 -> BitOut/1
  Constant4/1 -> Relational Operator/2
  Constant2/1 -> Shift Arithmetic/1
  Bitwise Operator/1 -> Relational Operator/1
  U/1 -> Bitwise Operator/1
  Shift Arithmetic/1 -> Bitwise Operator/2
  Bit/1 -> Shift Arithmetic/2

== system MdXX_RspOutComm/MdXX_RspOutCommCalc_Cal_sys/Subsystem/MdRspOutDataSelc31/BitSelector1 ==
  U : Inport
  Bit : Inport  Port=2
  Bitwise Operator : simulink/Logic and Bit Operations/Bitwise Operator  logicop=AND  UseBitMask=off  NumInputPorts=2  BitMask=bin2dec('11011001')  BitMaskRealWorld=Stored Integer
  Constant2 : Constant  OutDataTypeStr=uint32
  Constant4 : Constant  Value=0  OutDataTypeStr=uint32
  Relational Operator : RelationalOperator  Operator=>  OutDataTypeStr=boolean  RndMeth=Simplest  InputSameDT=off
  Shift Arithmetic : ArithShift  BitShiftNumberSource=Input port  BitShiftNumber=8  BitShiftDirection=Left
      settings: InputPortMap=u0,p1
  BitOut : Outport  VectorParamsAs1DForOutWhenUnconnected=off
  wires:
  Bit/1 -> Shift Arithmetic/2
  Shift Arithmetic/1 -> Bitwise Operator/2
  U/1 -> Bitwise Operator/1
  Bitwise Operator/1 -> Relational Operator/1
  Constant2/1 -> Shift Arithmetic/1
  Constant4/1 -> Relational Operator/2
  Relational Operator/1 -> BitOut/1

== system MdXX_RspOutComm/MdXX_RspOutCommCalc_Cal_sys/Subsystem/MdRspOutDataSelc32/BitSelector ==
  U : Inport
  Bit : Inport  Port=2
  Bitwise Operator : simulink/Logic and Bit Operations/Bitwise Operator  logicop=AND  UseBitMask=off  NumInputPorts=2  BitMask=bin2dec('11011001')  BitMaskRealWorld=Stored Integer
  Constant2 : Constant  OutDataTypeStr=uint32
  Constant4 : Constant  Value=0  OutDataTypeStr=uint32
  Relational Operator : RelationalOperator  Operator=>  OutDataTypeStr=boolean  RndMeth=Simplest  InputSameDT=off
  Shift Arithmetic : ArithShift  BitShiftNumberSource=Input port  BitShiftNumber=8  BitShiftDirection=Left
      settings: InputPortMap=u0,p1
  BitOut : Outport  VectorParamsAs1DForOutWhenUnconnected=off
  wires:
  Bit/1 -> Shift Arithmetic/2
  Shift Arithmetic/1 -> Bitwise Operator/2
  U/1 -> Bitwise Operator/1
  Bitwise Operator/1 -> Relational Operator/1
  Constant2/1 -> Shift Arithmetic/1
  Constant4/1 -> Relational Operator/2
  Relational Operator/1 -> BitOut/1

== system MdXX_RspOutComm/MdXX_RspOutCommCalc_Cal_sys/Subsystem/MdRspOutDataSelc32/BitSelector1 ==
  U : Inport
  Bit : Inport  Port=2
  Bitwise Operator : simulink/Logic and Bit Operations/Bitwise Operator  logicop=AND  UseBitMask=off  NumInputPorts=2  BitMask=bin2dec('11011001')  BitMaskRealWorld=Stored Integer
  Constant2 : Constant  OutDataTypeStr=uint32
  Constant4 : Constant  Value=0  OutDataTypeStr=uint32
  Relational Operator : RelationalOperator  Operator=>  OutDataTypeStr=boolean  RndMeth=Simplest  InputSameDT=off
  Shift Arithmetic : ArithShift  BitShiftNumberSource=Input port  BitShiftNumber=8  BitShiftDirection=Left
      settings: InputPortMap=u0,p1
  BitOut : Outport  VectorParamsAs1DForOutWhenUnconnected=off
  wires:
  Relational Operator/1 -> BitOut/1
  Constant4/1 -> Relational Operator/2
  Constant2/1 -> Shift Arithmetic/1
  Bitwise Operator/1 -> Relational Operator/1
  U/1 -> Bitwise Operator/1
  Shift Arithmetic/1 -> Bitwise Operator/2
  Bit/1 -> Shift Arithmetic/2

== system MdXX_RspOutComm/MdXX_RspOutCommCalc_Cal_sys/Subsystem/MdRspOutDataSelc4/BitSelector ==
  U : Inport
  Bit : Inport  Port=2
  Bitwise Operator : simulink/Logic and Bit Operations/Bitwise Operator  logicop=AND  UseBitMask=off  NumInputPorts=2  BitMask=bin2dec('11011001')  BitMaskRealWorld=Stored Integer
  Constant2 : Constant  OutDataTypeStr=uint32
  Constant4 : Constant  Value=0  OutDataTypeStr=uint32
  Relational Operator : RelationalOperator  Operator=>  OutDataTypeStr=boolean  RndMeth=Simplest  InputSameDT=off
  Shift Arithmetic : ArithShift  BitShiftNumberSource=Input port  BitShiftNumber=8  BitShiftDirection=Left
      settings: InputPortMap=u0,p1
  BitOut : Outport  VectorParamsAs1DForOutWhenUnconnected=off
  wires:
  Bit/1 -> Shift Arithmetic/2
  Shift Arithmetic/1 -> Bitwise Operator/2
  U/1 -> Bitwise Operator/1
  Bitwise Operator/1 -> Relational Operator/1
  Constant2/1 -> Shift Arithmetic/1
  Constant4/1 -> Relational Operator/2
  Relational Operator/1 -> BitOut/1

== system MdXX_RspOutComm/MdXX_RspOutCommCalc_Cal_sys/Subsystem/MdRspOutDataSelc4/BitSelector1 ==
  U : Inport
  Bit : Inport  Port=2
  Bitwise Operator : simulink/Logic and Bit Operations/Bitwise Operator  logicop=AND  UseBitMask=off  NumInputPorts=2  BitMask=bin2dec('11011001')  BitMaskRealWorld=Stored Integer
  Constant2 : Constant  OutDataTypeStr=uint32
  Constant4 : Constant  Value=0  OutDataTypeStr=uint32
  Relational Operator : RelationalOperator  Operator=>  OutDataTypeStr=boolean  RndMeth=Simplest  InputSameDT=off
  Shift Arithmetic : ArithShift  BitShiftNumberSource=Input port  BitShiftNumber=8  BitShiftDirection=Left
      settings: InputPortMap=u0,p1
  BitOut : Outport  VectorParamsAs1DForOutWhenUnconnected=off
  wires:
  Relational Operator/1 -> BitOut/1
  Constant4/1 -> Relational Operator/2
  Constant2/1 -> Shift Arithmetic/1
  Bitwise Operator/1 -> Relational Operator/1
  U/1 -> Bitwise Operator/1
  Shift Arithmetic/1 -> Bitwise Operator/2
  Bit/1 -> Shift Arithmetic/2

== system MdXX_RspOutComm/MdXX_RspOutCommCalc_Cal_sys/Subsystem/MdRspOutDataSelc5/BitSelector ==
  U : Inport
  Bit : Inport  Port=2
  Bitwise Operator : simulink/Logic and Bit Operations/Bitwise Operator  logicop=AND  UseBitMask=off  NumInputPorts=2  BitMask=bin2dec('11011001')  BitMaskRealWorld=Stored Integer
  Constant2 : Constant  OutDataTypeStr=uint32
  Constant4 : Constant  Value=0  OutDataTypeStr=uint32
  Relational Operator : RelationalOperator  Operator=>  OutDataTypeStr=boolean  RndMeth=Simplest  InputSameDT=off
  Shift Arithmetic : ArithShift  BitShiftNumberSource=Input port  BitShiftNumber=8  BitShiftDirection=Left
      settings: InputPortMap=u0,p1
  BitOut : Outport  VectorParamsAs1DForOutWhenUnconnected=off
  wires:
  Relational Operator/1 -> BitOut/1
  Constant4/1 -> Relational Operator/2
  Constant2/1 -> Shift Arithmetic/1
  Bitwise Operator/1 -> Relational Operator/1
  U/1 -> Bitwise Operator/1
  Shift Arithmetic/1 -> Bitwise Operator/2
  Bit/1 -> Shift Arithmetic/2

== system MdXX_RspOutComm/MdXX_RspOutCommCalc_Cal_sys/Subsystem/MdRspOutDataSelc5/BitSelector1 ==
  U : Inport
  Bit : Inport  Port=2
  Bitwise Operator : simulink/Logic and Bit Operations/Bitwise Operator  logicop=AND  UseBitMask=off  NumInputPorts=2  BitMask=bin2dec('11011001')  BitMaskRealWorld=Stored Integer
  Constant2 : Constant  OutDataTypeStr=uint32
  Constant4 : Constant  Value=0  OutDataTypeStr=uint32
  Relational Operator : RelationalOperator  Operator=>  OutDataTypeStr=boolean  RndMeth=Simplest  InputSameDT=off
  Shift Arithmetic : ArithShift  BitShiftNumberSource=Input port  BitShiftNumber=8  BitShiftDirection=Left
      settings: InputPortMap=u0,p1
  BitOut : Outport  VectorParamsAs1DForOutWhenUnconnected=off
  wires:
  Bit/1 -> Shift Arithmetic/2
  Shift Arithmetic/1 -> Bitwise Operator/2
  U/1 -> Bitwise Operator/1
  Bitwise Operator/1 -> Relational Operator/1
  Constant2/1 -> Shift Arithmetic/1
  Constant4/1 -> Relational Operator/2
  Relational Operator/1 -> BitOut/1

== system MdXX_RspOutComm/MdXX_RspOutCommCalc_Cal_sys/Subsystem/MdRspOutDataSelc6/BitSelector ==
  U : Inport
  Bit : Inport  Port=2
  Bitwise Operator : simulink/Logic and Bit Operations/Bitwise Operator  logicop=AND  UseBitMask=off  NumInputPorts=2  BitMask=bin2dec('11011001')  BitMaskRealWorld=Stored Integer
  Constant2 : Constant  OutDataTypeStr=uint32
  Constant4 : Constant  Value=0  OutDataTypeStr=uint32
  Relational Operator : RelationalOperator  Operator=>  OutDataTypeStr=boolean  RndMeth=Simplest  InputSameDT=off
  Shift Arithmetic : ArithShift  BitShiftNumberSource=Input port  BitShiftNumber=8  BitShiftDirection=Left
      settings: InputPortMap=u0,p1
  BitOut : Outport  VectorParamsAs1DForOutWhenUnconnected=off
  wires:
  Bit/1 -> Shift Arithmetic/2
  Shift Arithmetic/1 -> Bitwise Operator/2
  U/1 -> Bitwise Operator/1
  Bitwise Operator/1 -> Relational Operator/1
  Constant2/1 -> Shift Arithmetic/1
  Constant4/1 -> Relational Operator/2
  Relational Operator/1 -> BitOut/1
